simulink model "Simulacao2MA"  (R2023b)
settings: Solver=VariableStepAuto  StartTime=0.0  StopTime=2  RelTol=1e-3
undefined symbols (not defined in the file or in its folder): C, d, den, L, num, R, Tpwm, Vs
libraries: spsSeriesRLCBranchLib x3, spsCurrentMeasurementLib x1, spsDCVoltageSourceLib x1, spsDiodeLib x1, spsGroundLib x1, simulink x1, spsMosfetLib x1, commseqgen3 x1, spsVoltageMeasurementLib x1, sps_lib x1
settings Model: Creator=luisf  LastModifiedBy=luisf

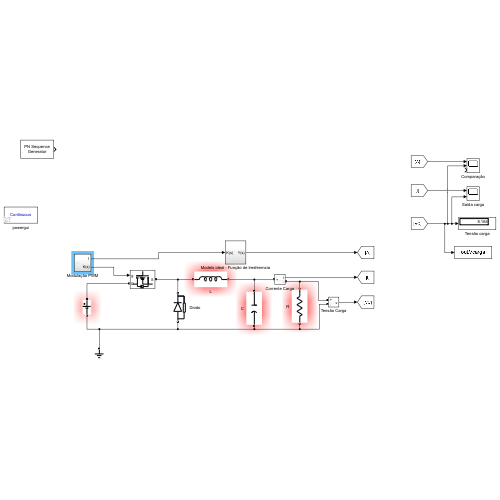
[thumbnail: Simulink's stored preview of the top-level diagram]
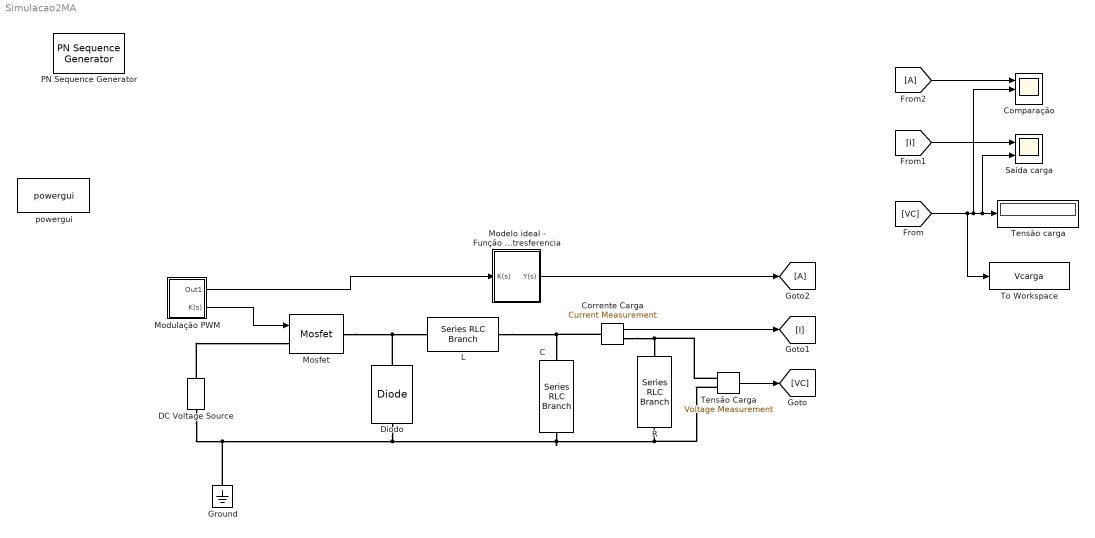
== system Simulacao2MA ==
  C : spsSeriesRLCBranchLib/Series RLC Branch  LConnTagsString=__new0  RConnTagsString=__new0  BranchType=C  Resistance=1  Inductance=1e-3  SetiL0=off  InitialCurrent=0  Capacitance=C  Setx0=off  InitialVoltage=0  Measurements=None
  Comparação : Scope  NumInputPorts=3
  Corrente Carga : spsCurrentMeasurementLib/Current Measurement  PhasorSimulation=off  OutputType=Complex  PSBequivalent=0
  DC Voltage Source : spsDCVoltageSourceLib/DC Voltage Source  Amplitude=Vs  Measurements=None
  Diodo : spsDiodeLib/Diode  Ron=0.0001  Lon=0  Vf=0.8  IC=0  UseSnubber=0  Rs=500  Cs=250e-9  Measurements=off
  From2 : From
  Goto2 : Goto
  Ground : spsGroundLib/Ground  LConnTagsString=a
  L : spsSeriesRLCBranchLib/Series RLC Branch  LConnTagsString=__new0  RConnTagsString=__new0  BranchType=L  Resistance=1  Inductance=L  SetiL0=off  InitialCurrent=0  Capacitance=1e-6  Setx0=off  InitialVoltage=0  Measurements=None
  Modelo ideal - Função de tresferencia : Subsystem
  Modulação PWM : Subsystem
  Mosfet : spsMosfetLib/Mosfet  Ron=0.1  Lon=0  Rd=0.01  Vfd=0  IC=0  Rs=1e5  Cs=inf  Measurements=off
  PN Sequence Generator : commseqgen3/PN Sequence Generator  poly=[15 14 0]  ini_sta=ones(1, 15)  outBitMaskSource=Dialog parameter  shift=0  outVarSiz=off  maxOutSizeMode=Dialog parameter  maxOutSize=[10 1]  Ts=Tpwm  sampPerFrame=1  reset=off  bitPackedOutputs=off  outDataType=double  numPackedBits=8  bitPackDataSigned=off  bitPackedOutDType=double
  R : spsSeriesRLCBranchLib/Series RLC Branch  LConnTagsString=__new0  RConnTagsString=__new0  BranchType=R  Resistance=R  Inductance=1e-3  SetiL0=off  InitialCurrent=0  Capacitance=1e-6  Setx0=off  InitialVoltage=0  Measurements=None
  Saída carga : Scope  NumInputPorts=2
  Tensão Carga : spsVoltageMeasurementLib/Voltage Measurement  PhasorSimulation=off  OutputType=Complex  PSBequivalent=0
  Tensão carga : Display
  To Workspace : ToWorkspace  VariableName=Vcarga  SampleTime=-1
  powergui : sps_lib/powergui  Priority=1  SimulationMode=Continuous  SampleTime=50e-6  frequency=60  Iterations=50  frequencyindice=0  Pbase=100e6  ErrMax=1e-4  UnitsV=kV  UnitsW=MW  buscounter=0  FunctionMessages=off  echomessages=off  EnableUseOfTLC=off  CurrentSourceSwitches=off  DisableSnubberDevices=off  DisableRonSwitches=off  DisableVfSwitches=off  DisplayEquations=off  AutomaticDiscreteSolvers=off  SolverType=Tustin/Backward Euler (TBE)  Interpol=off  ExternalGateDelay=off  methode=off  Ts=100  x0status=blocks  SPID=on  SwTol=0  HookPort=off  NonlinearTolerance=1e-4  nMaxIteration=100  ContinueOnMaxIteration=off  RestoreLinks=warning  ResistiveCurrentMeasurement=off  Frange=[0:2:500]  Ylog=off  Xlog=on  ShowGrid=off  save=off  variable=ZData  structure=0  ZoomFFT=off  StartTime=0.0  cycles=1  DisplayStyle=1  fundamental=60  FreqAxis=off  MaxFrequency=1000  frequencyindicesteady=1  RmsSteady=1  display=off
  wires:
  Tensão Carga/1 -> [VC]
  Corrente Carga/1 -> [I]
  [VC] -> To Workspace/1, Comparação/2, Saída carga/2, Tensão carga/1
  [I] -> Saída carga/1
  Modelo ideal - Função de tresferencia/1(Y(s)) -> Goto2/1
  From2/1 -> Comparação/1
  Modulação PWM/2(K(s)) -> Mosfet/1
  Modulação PWM/1(Out1) -> Modelo ideal - Função de tresferencia/1(K(s))
  connections:
  DC Voltage Source/RConn1 -- Mosfet/LConn1
  Mosfet/RConn1 -- Diodo/RConn1 -- L/LConn1
  L/RConn1 -- Corrente Carga/LConn1 -- C/LConn1
  DC Voltage Source/LConn1 -- Ground/LConn1 -- Diodo/LConn1 -- C/RConn1 -- Tensão Carga/LConn2 -- R/RConn1
  Tensão Carga/LConn1 -- Corrente Carga/RConn1 -- R/LConn1

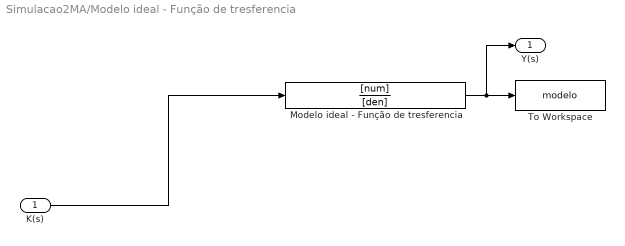
== system Simulacao2MA/Modelo ideal - Função de tresferencia ==
  K(s) : Inport
  Modelo ideal - Função de tresferencia : TransferFcn  Numerator=[num]  Denominator=[den]
  To Workspace : ToWorkspace  VariableName=modelo  SampleTime=-1
  Y(s) : Outport
  wires:
  Modelo ideal - Função de tresferencia/1 -> Y(s)/1, To Workspace/1
  K(s)/1 -> Modelo ideal - Função de tresferencia/1

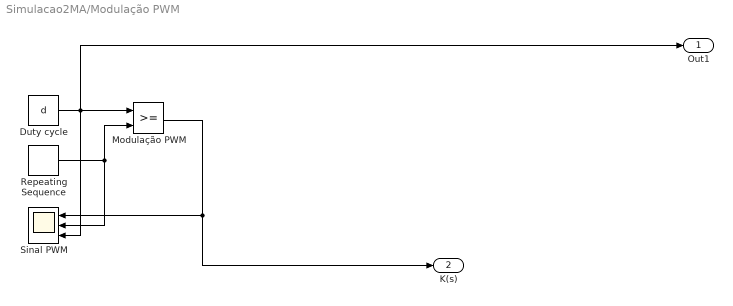
== system Simulacao2MA/Modulação PWM ==
  Duty cycle : Constant  Value=d
  Modulação PWM : RelationalOperator  OutDataTypeStr=boolean  RndMeth=Simplest  InputSameDT=off
  Repeating Sequence : simulink/Sources/Repeating Sequence  rep_seq_t=[0 Tpwm]  rep_seq_y=[0 1]
  Sinal PWM : Scope  NumInputPorts=3
  Out1 : Outport
  K(s) : Outport  Port=2  OutDataTypeStr=boolean
  wires:
  Repeating Sequence/1 -> Sinal PWM/2, Modulação PWM/2
  Modulação PWM/1 -> K(s)/1, Sinal PWM/1
  Duty cycle/1 -> Out1/1, Modulação PWM/1, Sinal PWM/3
